simulink model "Problem3"  (R2020a)
settings: Solver=VariableStepAuto  StartTime=0.0  StopTime=10.0  RelTol=1e-3
model workspace (MAT data in the model file):
  f = 200
settings Model: Creator=tnradm  LastModifiedBy=tnradm

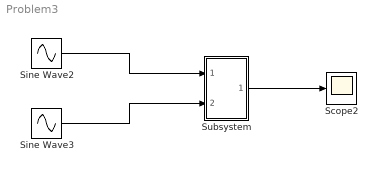
== system Problem3 ==
  Scope2 : Scope
  Sine Wave2 : Sin  SampleTime=0
  Sine Wave3 : Sin  SampleTime=0
  Subsystem : Subsystem
  wires:
  Sine Wave2/1 -> Subsystem/1(In1)
  Sine Wave3/1 -> Subsystem/2(In2)
  Subsystem/1(Out1) -> Scope2/1

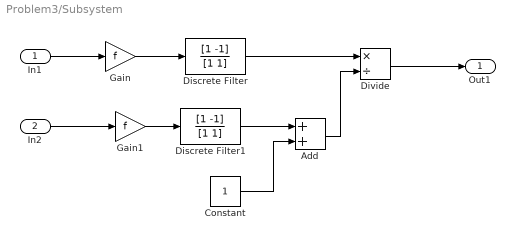
== system Problem3/Subsystem ==
  In1 : Inport
  In2 : Inport  Port=2
  Add : Sum
  Constant : Constant
  Discrete Filter : DiscreteFilter  Numerator=[1 -1]  Denominator=[1 1]
  Discrete Filter1 : DiscreteFilter  Numerator=[1 -1]  Denominator=[1 1]
  Divide : Product  Inputs=*/
  Gain : Gain  Gain=f
  Gain1 : Gain  Gain=f
  Out1 : Outport
  wires:
  In2/1 -> Gain1/1
  Divide/1 -> Out1/1
  Gain1/1 -> Discrete Filter1/1
  Add/1 -> Divide/2
  Discrete Filter/1 -> Divide/1
  Gain/1 -> Discrete Filter/1
  In1/1 -> Gain/1
  Constant/1 -> Add/2
  Discrete Filter1/1 -> Add/1
